simulink model "lista1_2b"  (R2020b)
settings: Solver=VariableStepAuto  StartTime=0.0  StopTime=10  RelTol=1e-3
settings Model: Creator=lucas  LastModifiedBy=lucas

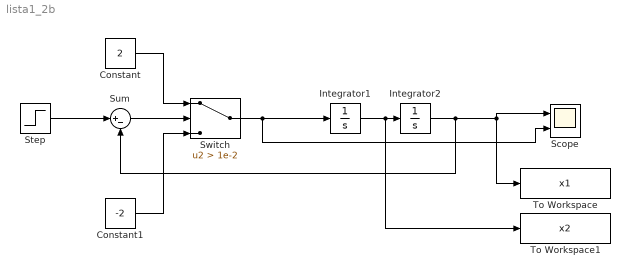
== system lista1_2b ==
  Constant : Constant  Value=2
  Constant1 : Constant  Value=-2
  Integrator1 : Integrator
  Integrator2 : Integrator
  Scope : Scope  NumInputPorts=2
  Step : Step  Time=0  SampleTime=0
  Sum : Sum  Inputs=|+-
  Switch : Switch  Criteria=u2 > Threshold  Threshold=1e-2
  To Workspace : ToWorkspace  VariableName=x1  SaveFormat=Timeseries  SampleTime=-1
  To Workspace1 : ToWorkspace  VariableName=x2  SaveFormat=Timeseries  SampleTime=-1
  wires:
  Step/1 -> Sum/1
  Sum/1 -> Switch/2
  Integrator1/1 -> To Workspace1/1, Integrator2/1
  Switch/1 -> Scope/2, Integrator1/1
  Constant/1 -> Switch/1
  Constant1/1 -> Switch/3
  Integrator2/1 -> To Workspace/1, Scope/1, Sum/2
